simulink model "DAEbot_model"  (R2018a)
settings: Solver=FixedStepDiscrete  StartTime=0.0  StopTime=inf  RelTol=1e-3  EnableMultiTasking=on
undefined symbols (not defined in the file): Mag_Thresh, Mode, SafeAtSide_Thresh, SafeInFrnt_Thresh, UnInit
libraries: simulink x19
settings Model: Creator=uwlau  LastModifiedBy=Mangal
settings SolverCC: PositivePriorityOrder=on  AutoInsertRateTranBlk=on
settings OptimizationCC: DefaultParameterBehavior=Inlined  InlineInvariantSignals=on  EnhancedBackFolding=on  PassReuseOutputArgsAs=Individual arguments  StateBitsets=on  DataBitsets=on  ZeroExternalMemoryAtStartup=off  ZeroInternalMemoryAtStartup=off  NoFixptDivByZeroProtection=on  MaxStackSize=64  OptimizeBlockOrder=speed  DifferentSizesBufferReuse=on
settings DebuggingCC: ParameterTunabilityLossMsg=error
settings HardwareCC: ProdBitPerPointer=32  ProdBitPerSizeT=32  ProdBitPerPtrDiffT=32  ProdLargestAtomicInteger=Long  ProdLargestAtomicFloat=Double  ProdWordSize=32  ProdHWDeviceType=ARM Compatible->ARM Cortex
settings ModelReferenceCC: EnableParallelModelReferenceBuilds=on
settings SFSimCC: MATLABDynamicMemAlloc=off
settings RTWCC: SystemTargetFile=ert.tlc  HardwareBoard=Raspberry Pi  TLCOptions=-p0 -aRateBasedStepFcn=0  TemplateMakefile=ert_default_tmf  GenerateReport=on  CustomHeaderCode="#include \"MQTT_Subscriber.h\""  CustomInclude=../../../../Peripheral-Drivers/DAEbot-PD/MQTT/mqtt_lib ../../../../Peripheral-Drivers/DAEbot-PD/MQTT/paho_mqtt_headers ../../../../Peripheral-Drivers/DAEbot-PD/MQTT/paho_bin  CustomSource=../../../../Peripheral-Drivers/DAEbot-PD/MQTT/mqtt_lib/MQTT_Subscriber.c  Toolchain=GNU GCC Raspberry Pi  BuildConfiguration=Specify  IncludeHyperlinkInReport=on  LaunchReport=on  GenerateTraceInfo=on  GenerateTraceReport=on  GenerateTraceReportSl=on  GenerateTraceReportSf=on  GenerateTraceReportEml=on
settings CodeAppCC: ForceParamTrailComments=on  IgnoreCustomStorageClasses=off  OperatorAnnotations=on  SimulinkDataObjDesc=on  SFDataObjDesc=on  InsertBlockDesc=on
settings ERTTargetCC: InlinedParameterPlacement=NonHierarchical  ERTCustomFileTemplate=example_file_process.tlc

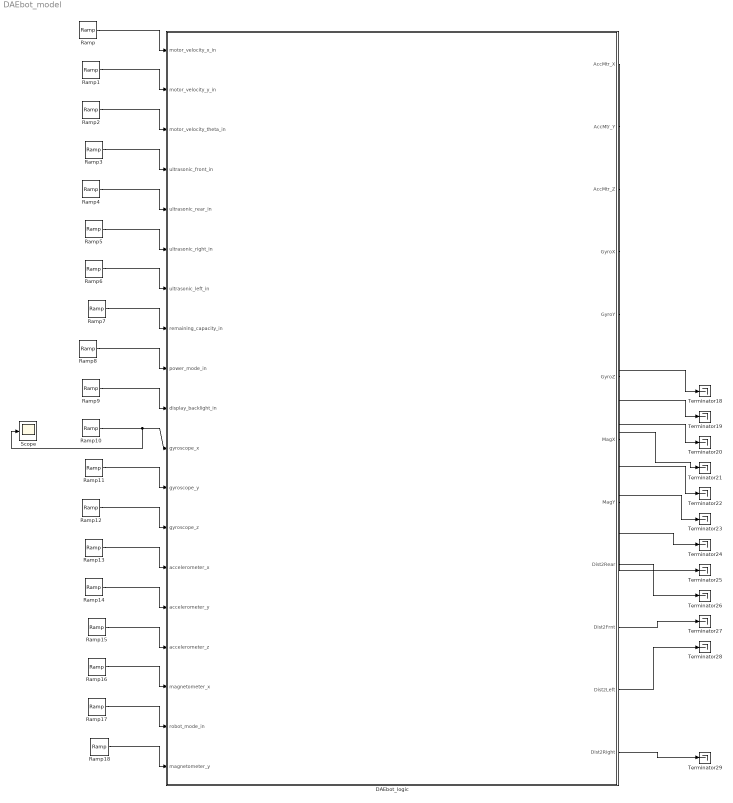
== system DAEbot_model ==
  DAEbot_logic : Stateflow chart  TreatAsAtomicUnit=on
  Ramp{,1..18} (19 alike) : simulink/Sources/Ramp  slope=1  start=0  InitialOutput=0
  Scope : Scope
  Terminator{18..29} (12 alike) : Terminator
  wires:
  Ramp/1 -> DAEbot_logic/1(motor_velocity_x_in)
  Ramp1/1 -> DAEbot_logic/2(motor_velocity_y_in)
  Ramp3/1 -> DAEbot_logic/4(ultrasonic_front_in)
  Ramp2/1 -> DAEbot_logic/3(motor_velocity_theta_in)
  Ramp6/1 -> DAEbot_logic/7(ultrasonic_left_in)
  Ramp7/1 -> DAEbot_logic/8(remaining_capacity_in)
  Ramp5/1 -> DAEbot_logic/6(ultrasonic_right_in)
  Ramp4/1 -> DAEbot_logic/5(ultrasonic_rear_in)
  Ramp12/1 -> DAEbot_logic/13(gyroscope_z)
  Ramp13/1 -> DAEbot_logic/14(accelerometer_x)
  Ramp15/1 -> DAEbot_logic/16(accelerometer_z)
  Ramp14/1 -> DAEbot_logic/15(accelerometer_y)
  Ramp11/1 -> DAEbot_logic/12(gyroscope_y)
  Ramp9/1 -> DAEbot_logic/10(display_backlight_in)
  Ramp8/1 -> DAEbot_logic/9(power_mode_in)
  Ramp17/1 -> DAEbot_logic/18(robot_mode_in)
  Ramp18/1 -> DAEbot_logic/19(magnetometer_y)
  Ramp16/1 -> DAEbot_logic/17(magnetometer_x)
  DAEbot_logic/1(AccMtr_X) -> Terminator18/1
  DAEbot_logic/2(AccMtr_Y) -> Terminator19/1
  DAEbot_logic/4(GyroX) -> Terminator21/1
  DAEbot_logic/3(AccMtr_Z) -> Terminator20/1
  DAEbot_logic/7(MagX) -> Terminator24/1
  DAEbot_logic/8(MagY) -> Terminator25/1
  DAEbot_logic/6(GyroZ) -> Terminator23/1
  DAEbot_logic/5(GyroY) -> Terminator22/1
  DAEbot_logic/9(Dist2Rear) -> Terminator26/1
  DAEbot_logic/12(Dist2Right) -> Terminator29/1
  DAEbot_logic/11(Dist2Left) -> Terminator28/1
  DAEbot_logic/10(Dist2Frnt) -> Terminator27/1
  Ramp10/1 -> Scope/1, DAEbot_logic/11(gyroscope_x)

== stateflow chart DAEbot_model/DAEbot_logic ==
  state Scanner
    state Motion_Detect [parallel]
      settings: executionOrder=1
      state MotionSet
        en:
        BotInAct = 1;
      state MotionNtSet
        en:
        BotInAct = 0;
      (default) -> MotionNtSet
      MotionNtSet -> MotionSet : [motor_velocity_x_in||motor_velocity_x_in||motor_velocity_x_in]
      MotionSet -> MotionNtSet : [motor_velocity_x_in == 0&&motor_velocity_y_in==0&&motor_velocity_theta_in==0]
    state Accmtr [parallel]
      settings: executionOrder=4
      state gyro_X [parallel]
        settings: executionOrder=1
        state gyro_X_Set
          en:
          AccMtr_X =accelerometer_x;
        state gyro_X_Init
          en:
          AccMtr_X = UnInit;
        Scanner.Accmtr.gyro_X.gyro_X_Init -> Scanner.Accmtr.gyro_X.gyro_X_Set : [ultrasonic_front_in ~=0]
        (default) -> Scanner.Accmtr.gyro_X.gyro_X_Init
        Scanner.Accmtr.gyro_X.gyro_X_Set -> Scanner.Accmtr.gyro_X.gyro_X_Init : [ultrasonic_front_in == 0]
      state gyro_Y [parallel]
        settings: executionOrder=2
        state gyro_Y_Init1
          en:
          AccMtr_Y =accelerometer_y;
        state gyro_Y_Init
          en:
          AccMtr_Y = UnInit;
        Scanner.Accmtr.gyro_Y.gyro_Y_Init -> Scanner.Accmtr.gyro_Y.gyro_Y_Init1 : [ultrasonic_front_in ~=0]
        (default) -> Scanner.Accmtr.gyro_Y.gyro_Y_Init
        Scanner.Accmtr.gyro_Y.gyro_Y_Init1 -> Scanner.Accmtr.gyro_Y.gyro_Y_Init : [ultrasonic_front_in == 0]
      state gyro_Z [parallel]
        settings: executionOrder=3
        state gyro_Z_Init1
          en:
          AccMtr_Z =accelerometer_z;
        state gyro_Z_Init
          en:
          AccMtr_Z = UnInit;
        Scanner.Accmtr.gyro_Z.gyro_Z_Init -> Scanner.Accmtr.gyro_Z.gyro_Z_Init1 : [ultrasonic_front_in ~=0]
        (default) -> Scanner.Accmtr.gyro_Z.gyro_Z_Init
        Scanner.Accmtr.gyro_Z.gyro_Z_Init1 -> Scanner.Accmtr.gyro_Z.gyro_Z_Init : [ultrasonic_front_in == 0]
    state Ultrasonic [parallel]
      settings: executionOrder=2
      state Frnt [parallel]
        settings: executionOrder=1
        state Frnt_set
          du:
          Dist2Frnt =ultrasonic_front_in;
        state Frnt_Uninit
          en:
          Dist2Frnt = UnInit;
        Frnt_Uninit -> Frnt_set : [BotInAct && ultrasonic_front_in ~=0]
        (default) -> Frnt_Uninit
        Frnt_set -> Frnt_Uninit : [ultrasonic_front_in == 0]
      state Back [parallel]
        settings: executionOrder=2
        state Rear_Set
          du:
          Dist2Rear =ultrasonic_rear_in;
        state Rear_Uninit
          en:
          Dist2Rear= UnInit;
        Rear_Uninit -> Rear_Set : [BotInAct && ultrasonic_rear_in ~=0]
        (default) -> Rear_Uninit
        Rear_Set -> Rear_Uninit : [ultrasonic_rear_in == 0]
      state Left [parallel]
        settings: executionOrder=3
        state Left_Set
          du:
          Dist2Left =ultrasonic_left_in;
        state Left_Uninit
          en:
          Dist2Left = UnInit;
        Left_Uninit -> Left_Set : [BotInAct && ultrasonic_left_in ~=0]
        (default) -> Left_Uninit
        Left_Set -> Left_Uninit : [ultrasonic_left_in == 0]
      state Right [parallel]
        settings: executionOrder=4
        state Right_Set
          du:
          Dist2Right =ultrasonic_right_in;
        state Right_Uninit
          en:
          Dist2Right = UnInit;
        Right_Uninit -> Right_Set : [BotInAct && ultrasonic_right_in ~=0]
        (default) -> Right_Uninit
        Right_Set -> Right_Uninit : [ultrasonic_right_in == 0]
    state gyro [parallel]
      settings: executionOrder=3
      state gyro_X [parallel]
        settings: executionOrder=1
        state gyro_X_Set
          en:
          GyroX =gyroscope_x;
        state gyro_X_Init
          en:
          GyroX = UnInit;
        Scanner.gyro.gyro_X.gyro_X_Init -> Scanner.gyro.gyro_X.gyro_X_Set : [ultrasonic_front_in ~=0]
        (default) -> Scanner.gyro.gyro_X.gyro_X_Init
        Scanner.gyro.gyro_X.gyro_X_Set -> Scanner.gyro.gyro_X.gyro_X_Init : [ultrasonic_front_in == 0]
      state gyro_Y [parallel]
        settings: executionOrder=2
        state gyro_Y_Init1
          en:
          GyroY =gyroscope_y;
        state gyro_Y_Init
          en:
          GyroY = UnInit;
        Scanner.gyro.gyro_Y.gyro_Y_Init -> Scanner.gyro.gyro_Y.gyro_Y_Init1 : [ultrasonic_front_in ~=0]
        (default) -> Scanner.gyro.gyro_Y.gyro_Y_Init
        Scanner.gyro.gyro_Y.gyro_Y_Init1 -> Scanner.gyro.gyro_Y.gyro_Y_Init : [ultrasonic_front_in == 0]
      state gyro_Z [parallel]
        settings: executionOrder=3
        state gyro_Z_Init1
          en:
          GyroZ =gyroscope_z;
        state gyro_Z_Init
          en:
          GyroZ = UnInit;
        Scanner.gyro.gyro_Z.gyro_Z_Init -> Scanner.gyro.gyro_Z.gyro_Z_Init1 : [ultrasonic_front_in ~=0]
        (default) -> Scanner.gyro.gyro_Z.gyro_Z_Init
        Scanner.gyro.gyro_Z.gyro_Z_Init1 -> Scanner.gyro.gyro_Z.gyro_Z_Init : [ultrasonic_front_in == 0]
    state MagnetoMeter [parallel]
      settings: executionOrder=5
      state Mag_X [parallel]
        settings: executionOrder=1
        state Mag_X_Set
          en:
          MagX =magnetometer_x;
        state Mag_X_Init
          en:
          MagX = UnInit;
        Mag_X_Init -> Mag_X_Set : [ultrasonic_front_in ~=0]
        (default) -> Mag_X_Init
        Mag_X_Set -> Mag_X_Init : [ultrasonic_front_in == 0]
      state Mag_Y [parallel]
        settings: executionOrder=2
        state Mag_Y_Set
          en:
          MagY =magnetometer_y;
        state Mag_Y_Init
          en:
          MagY = UnInit;
        Mag_Y_Init -> Mag_Y_Set : [ultrasonic_front_in ~=0]
        (default) -> Mag_Y_Init
        Mag_Y_Set -> Mag_Y_Init : [ultrasonic_front_in == 0]
    state Plot [parallel]
      en:
      c = 1;
      du:
      c = PlotBotMotion(c,Dist2Right,Dist2Right)
      v=calc_max_vel(7,7)
      settings: executionOrder=8
    state Motion_Control [parallel]
      settings: executionOrder=6
      state Motion_Longitudinal
      state Motion_Init
      state Motion_Lateral
      state Stepbac
      Motion_Longitudinal -> Motion_Longitudinal [order 1] : [Dist2Frnt > SafeInFrnt_Thresh]
      Motion_Init -> Motion_Longitudinal [order 1] : [magnetometer_x > Mag_Thresh &&...
          |  magnetometer_y < Mag_Thresh ]
      Motion_Longitudinal -> Motion_Init [order 2] : [Dist2Frnt < SafeInFrnt_Thresh]
      (default) -> Motion_Init
      Motion_Init -> Stepbac [order 3] : [after(5,sec)]
      Motion_Lateral -> Motion_Init [order 2] : [Dist2Left < SafeAtSide_Thresh &&...
          | Dist2Right < SafeAtSide_Thresh]
      Stepbac -> Motion_Init
      Motion_Init -> Motion_Lateral [order 2] : [magnetometer_x < Mag_Thresh &&...
          |  magnetometer_y > Mag_Thresh ]
      Motion_Lateral -> Motion_Lateral [order 1] : [Dist2Left > SafeAtSide_Thresh &&...
          | Dist2Right > SafeAtSide_Thresh]
    state Magnetometer_Decode [parallel]
      settings: executionOrder=7
  (default) -> Scanner
  data: vel_in function_input; ultrasonic_distance function_input; velocity function_output; calc1 function_input; X function_input; Y function_input; calc2 function_output; motor_velocity_x_in input; motor_velocity_y_in input; motor_velocity_theta_in input; ultrasonic_front_in input; ultrasonic_rear_in input; ultrasonic_right_in input; ultrasonic_left_in input; motor_velocity_y_tmp local int16; motor_velocity_x_tmp local int16; motor_velocity_theta_tmp local int16; remaining_capacity_in input; re_ca_counter local; re_ca_tmp local; power_mode_in input; power_mode_internal local; prev_power_mode_in local; display_backlight_in input; gyroscope_x input; gyroscope_y input; gyroscope_z input; accelerometer_x input; accelerometer_y input; accelerometer_z input; magnetometer_x input; robot_mode_in input; motor_velocity_y_to_tx local int16; motor_velocity_x_to_tx local int16; motor_velocity_theta_to_tx local int16; motor_velocity_y_auto local int16; motor_velocity_x_auto local int16; motor_velocity_theta_auto local int16; magnetometer_y input; UnInit parameter; SafeInFrnt_Thresh parameter; SafeAtSide_Thresh parameter; Mag_Thresh parameter; Mode parameter; AccMtr_X output; AccMtr_Y output; AccMtr_Z output; GyroX output; GyroY output; GyroZ output; MagX output; MagY output; Dist2Rear output; BotInAct local; Dist2Frnt output; Dist2Left output; Dist2Right output; v local; c local
  function velocity  = calc_max_vel(vel_in, ultrasonic_distance):
    | function velocity  = calc_max_vel(vel_in, ultrasonic_distance)
    | 
    | % velcity = vel_max / (distance_max - distance_min) * obstacle_distance;
    | calc = 100 / (0.8 - 0.2) * ultrasonic_distance;
    | velocity = calc;
    | 
    | % for negative axis
    | if(vel_in < 0)
    |     velocity = velocity * -1;
    |     
    |     % don't use max vel if input is smaller
    |     if (vel_in > velocity)
    |         velocity = vel_in;
    |     end   
    | 
    | elseif (vel_in > 0)
    |     % don't use max vel if input is smaller
    |     if (vel_in < velocity)
    |         velocity = vel_in;
    |     end
    | end
    | 
    | end
  function calc2 = PlotBotMotion(calc1,X,Y):
    | function calc2 = PlotBotMotion(calc1,X,Y)
    | %ax1 = subplot(2,1,1);
    | %ax2 = subplot(2,1,2);
    | 
    | disp("plottinh")
    | calc1 = X+Y;
    | figure;
    | hold on;
    | dx = 500;
    | Xrate = [];
    | Xrate = [Xrate X];
    | %Xrate(calc1) = X;
    | calc1 = calc1+1;
    |     plot(Xrate)
    |     
    | %axis(X,Y);
    | 
    | 
    | end
